simulink model "QCarModel_Excited"  (R2023b)
settings: Solver=FixedStepAuto  StartTime=0.0  StopTime=20.0  FixedStep=0.1  RelTol=1e-3
values from neighbouring files (symbols this model uses):
  c = 20000    [QCarModel_Frequency_V2.m]    (also in QCarModel_Parameters.m)
  d = 1500    [QCarModel_Frequency_V2.m]    (also in QCarModel_Parameters.m)
  m = mass(h)    [QCarModel_Frequency_V2.m]    (also in QCarModel_Parameters.m = 400)
settings Model: VariantFading=off  Creator=34140  LastModifiedBy=BeanieBabyJ

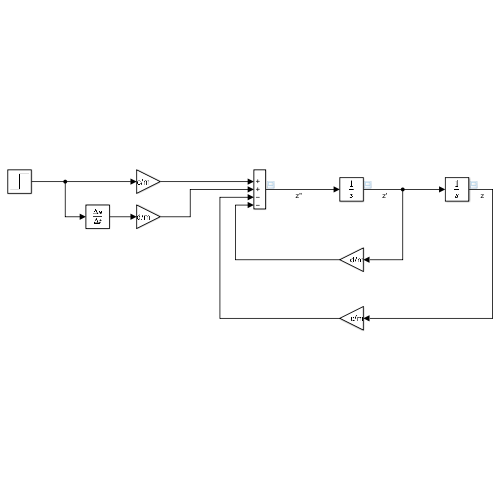
[thumbnail: Simulink's stored preview of the top-level diagram]
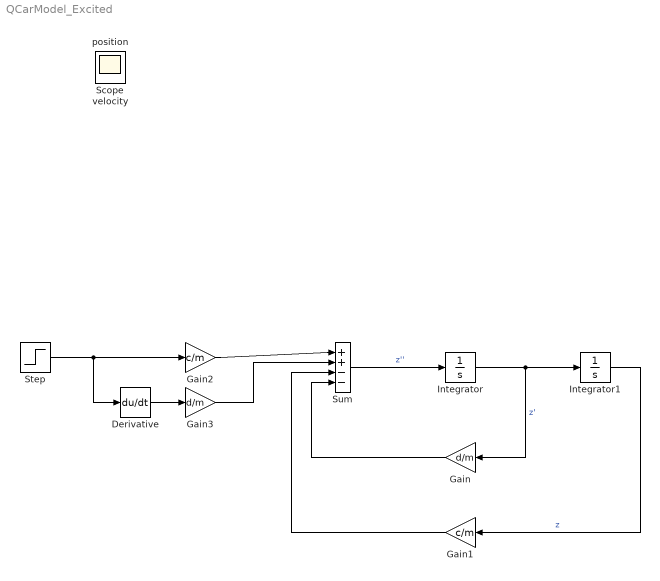
== system QCarModel_Excited ==
  Derivative : Derivative
  Gain : Gain  Gain=d/m
  Gain1 : Gain  Gain=c/m
  Gain2 : Gain  Gain=c/m
  Gain3 : Gain  Gain=d/m
  Integrator : Integrator
  Integrator1 : Integrator
  Step : Step  SampleTime=0
  Sum : Sum  Inputs=|++--
  Scope : Scope
  position : Scope
  velocity : Scope
  wires:
  Integrator/1 -> Gain/1, Integrator1/1  "z'"
  Sum/1 -> Integrator/1  "z''"
  Integrator1/1 -> Gain1/1  "z"
  Gain1/1 -> Sum/3
  Gain/1 -> Sum/4
  Derivative/1 -> Gain3/1
  Gain3/1 -> Sum/2
  Gain2/1 -> Sum/1
  Step/1 -> Derivative/1, Gain2/1
